simulink model "CNNPredict"  (R2024a)
settings: Solver=FixedStepAuto  StartTime=0.0  StopTime=inf  RelTol=1e-3  EnableMultiTasking=on
undefined symbols (not defined in the file or in its folder): Camera, Standard_Devices
libraries: pycoexlib x1, visionsinks x1, sldrtlib x1
settings Model: Creator=burli  LastModifiedBy=burli
settings SolverCC: AutoInsertRateTranBlk=on
settings OptimizationCC: EnhancedBackFolding=on  PassReuseOutputArgsThreshold=0  MaxStackSize=64  OptimizeBlockOrder=speed  DifferentSizesBufferReuse=on  OptimizationCustomize=off
settings DebuggingCC: ParameterTunabilityLossMsg=error
settings HardwareCC: ProdBitPerInt=16  ProdBitPerPointer=16  ProdBitPerSizeT=16  ProdBitPerPtrDiffT=16  ProdLargestAtomicFloat=None  ProdWordSize=8  ProdHWDeviceType=Atmel->AVR
settings SFSimCC: MATLABDynamicMemAlloc=off
settings RTWCC: Toolchain=Arduino AVR  BuildConfiguration=Faster Runs  GPUComputeCapability=3.5
settings CodeAppCC: ForceParamTrailComments=on  OperatorAnnotations=on
settings GRTTargetCC: TargetLangStandard=C89/C90 (ANSI)

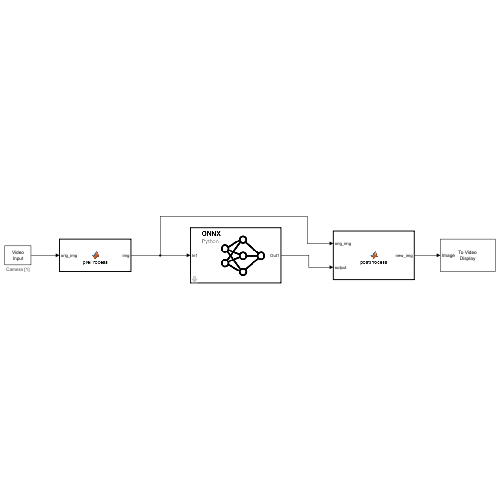
[thumbnail: Simulink's stored preview of the top-level diagram]
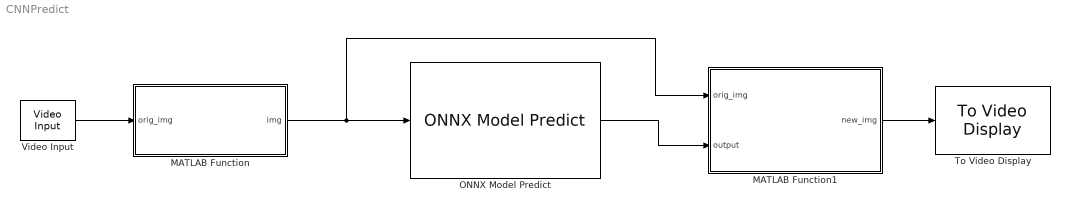
== system CNNPredict ==
  MATLAB Function : MATLAB Function  TreatAsAtomicUnit=on
  MATLAB Function1 : MATLAB Function  TreatAsAtomicUnit=on
  ONNX Model Predict : pycoexlib/ONNX Model Predict  ModelFile=C:\StewartProMatlab\SPro_Matlab_Mosfet v1_0_1\onnx_model_14.onnx  ExecutionProviders=CUDAExecutionProvider, CPUExecutionProvider  InputTable={ 'In1', 'float32', '[4 3 1 2]', 'inherit' }  OutputTable={ 'Out1', '', '' }  SampleTime=-1  InputDatatypes=float32  InputNumDims=inherit  InputPermutations=[4 3 1 2]  OutputPermutations=[]  PythonCoexecutionBlockType=ONNXModelBlock  VariableOutputMaxSizes=[]
  To Video Display : visionsinks/To Video Display  windowSizeMode=Normal  openAtMdlStart=on  fullScreen=off  videoWindowX=2056  videoWindowY=651  saveWindowSize=off  videoWindowWidth=320  videoWindowHeight=240  inputColorFormat=RGB  inputType=Obsolete  imagePorts=One multidimensional signal  OutputDevice=On-screen video monitor  dataOrg=Column-major  isWindowOpen=off
  Video Input : sldrtlib/Video Input  SampleTime=0.1  MaxMissedTicks=10  ShowMissedTicks=off  YieldWhenWaiting=off  DrvName=Standard_Devices/Camera  DrvAddress=1  DrvOptions=[320 240 1]  Channels=[1 2 3]  RoiOriginSource=1  RoiOrigin=[1 1]  RoiDimensions=[320 240]  ShowReady=off  ShowError=off  ShowTimestamp=off
      settings: AttributesFormatString=Camera [1]
  wires:
  Video Input/1 -> MATLAB Function/1(orig_img)
  MATLAB Function1/1(new_img) -> To Video Display/1
  MATLAB Function/1(img) -> MATLAB Function1/1(orig_img), ONNX Model Predict/1
  ONNX Model Predict/1 -> MATLAB Function1/2(output)

== matlab function CNNPredict/MATLAB Function ==
  data: orig_img input; img output
function img = preProcess(orig_img)
% 240,320,3
img=double(orig_img)/255.0;

== matlab function CNNPredict/MATLAB Function1 ==
  data: orig_img input; new_img output; output input
function new_img = postProcess(orig_img,output)

    orig_img = permute(orig_img,[3,1,2]);
    c = orig_img(1,:,:)+output;
    orig_img(1,:,:) = c./max(c,[],'all');

    orig_img = permute(orig_img,[2,3,1]);
    new_img = uint8(round(orig_img*255));
